simulink model "Yang2011"  (R2019a)
settings: Solver=VariableStepAuto  StartTime=0.0  StopTime=tsim  MaxStep=1e-3  RelTol=1e-12  EnableMultiTasking=on
values from neighbouring files (symbols this model uses):
  A = [a11 a12 0;a21 0 a23;0 a32 0]    [aa_MAGLEV_changeSlope.m]
  Ap = 0.01    [aa_MAGLEV_changeSlope.m]
  B1 = eye(3)    [aa_MAGLEV_changeSlope.m]
  B2 = [b2_11;0;0]    [aa_MAGLEV_changeSlope.m]
  G0 = 0.015    [aa_MAGLEV_changeSlope.m]
  I0 = (1/Kb)*B0*G0    [aa_MAGLEV_changeSlope.m]
  Kb = 0.0015    [aa_MAGLEV_changeSlope.m]
  KdY = -inv([0 0 1]*inv(A+B2*Kx)*B2)*[0 0 1]*inv(A+B2*Kx)*B1    [aa_MAGLEV_changeSlope.m]
  Kf = 9810    [aa_MAGLEV_changeSlope.m]
  KxY = Kx    [aa_MAGLEV_changeSlope.m]
  Lc = 0.1    [aa_MAGLEV_changeSlope.m]
  LY = [40 0 0 ... (first row only)    [aa_MAGLEV_changeSlope.m]
  mc = 1000    [aa_MAGLEV_changeSlope.m]
  Nc = 2000    [aa_MAGLEV_changeSlope.m]
  Rc = 10    [aa_MAGLEV_changeSlope.m]
  V0 = I0*Rc    [aa_MAGLEV_changeSlope.m]
settings Model: Creator=alcasfra  LastModifiedBy=alcas
settings SolverCC: AlgebraicLoopSolver=LineSearch
settings DataIOCC: ReturnWorkspaceOutputs=off
settings OptimizationCC: LifeSpan=inf
settings DebuggingCC: SFUnexpectedBacktrackingDiag=warning  SFNoUnconditionalDefaultTransitionDiag=warning  ArithmeticOperatorsInVariantConditions=warning
settings SFSimCC: SimUseLocalCustomCode=off
settings RTWCC: RTWUseLocalCustomCode=off
settings CodeAppCC: StateflowObjectComments=on
settings GRTTargetCC: TargetLangStandard=C89/C90 (ANSI)  GeneratePreprocessorConditionals=Disable all
settings ConfigComp: CovMetricSettings=dw  CovHtmlReporting=on  CovSaveCumulativeToWorkspaceVar=on  CovSaveSingleToWorkspaceVar=on  CovExternalEMLEnable=off

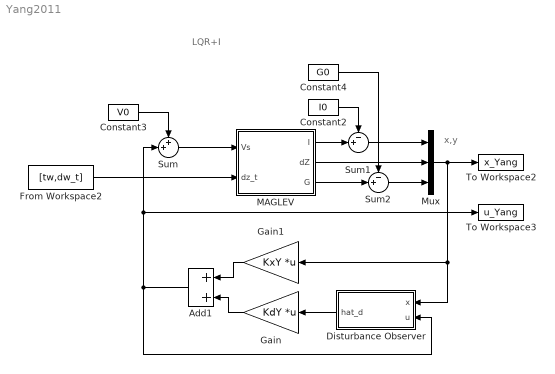
== system Yang2011 ==
  note: x,y
  note: LQR+I
  Add1 : Sum
  Constant2 : Constant  Value=I0
  Constant3 : Constant  Value=V0
  Constant4 : Constant  Value=G0
  Disturbance Observer : Subsystem
  From Workspace2 : FromWorkspace  VariableName=[tw,dw_t]  SampleTime=0
  Gain : Gain  Gain=KdY  Multiplication=Matrix(K*u)
  Gain1 : Gain  Gain=KxY  Multiplication=Matrix(K*u)
  MAGLEV : Subsystem
  Mux : Mux  Inputs=3
  Sum : Sum  Inputs=++|
  Sum1 : Sum  Inputs=-+|
  Sum2 : Sum  Inputs=-+|
  To Workspace2 : ToWorkspace  VariableName=x_Yang  SaveFormat=Structure With Time  SampleTime=-1
  To Workspace3 : ToWorkspace  VariableName=u_Yang  SaveFormat=Structure With Time  SampleTime=-1
  wires:
  Sum/1 -> MAGLEV/1(Vs)
  Constant3/1 -> Sum/1
  MAGLEV/1(I) -> Sum1/2
  Sum1/1 -> Mux/1
  MAGLEV/3(G) -> Sum2/2
  Sum2/1 -> Mux/3
  Constant2/1 -> Sum1/1
  Constant4/1 -> Sum2/1
  MAGLEV/2(dZ) -> Mux/2
  Mux/1 -> To Workspace2/1, Gain1/1, Disturbance Observer/1(x)
  Disturbance Observer/1(hat_d) -> Gain/1
  Gain1/1 -> Add1/1
  Gain/1 -> Add1/2
  Add1/1 -> Disturbance Observer/2(u), To Workspace3/1, Sum/2
  From Workspace2/1 -> MAGLEV/2(dz_t)

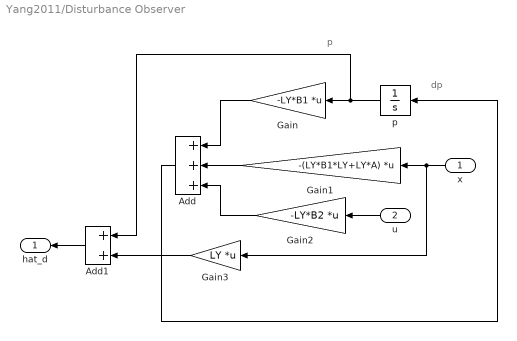
== system Yang2011/Disturbance Observer ==
  note: p
  note: dp
  x : Inport
  u : Inport  Port=2
  Add : Sum  Inputs=+++
  Add1 : Sum
  Gain : Gain  Gain=-LY*B1  Multiplication=Matrix(K*u)
  Gain1 : Gain  Gain=-(LY*B1*LY+LY*A)  Multiplication=Matrix(K*u)
  Gain2 : Gain  Gain=-LY*B2  Multiplication=Matrix(K*u)
  Gain3 : Gain  Gain=LY  Multiplication=Matrix(K*u)
  p : Integrator
  hat_d : Outport
  wires:
  x/1 -> Gain3/1, Gain1/1
  Gain2/1 -> Add/3
  u/1 -> Gain2/1
  Gain3/1 -> Add1/2
  Add1/1 -> hat_d/1
  Add/1 -> p/1
  Gain1/1 -> Add/2
  p/1 -> Add1/1, Gain/1
  Gain/1 -> Add/1

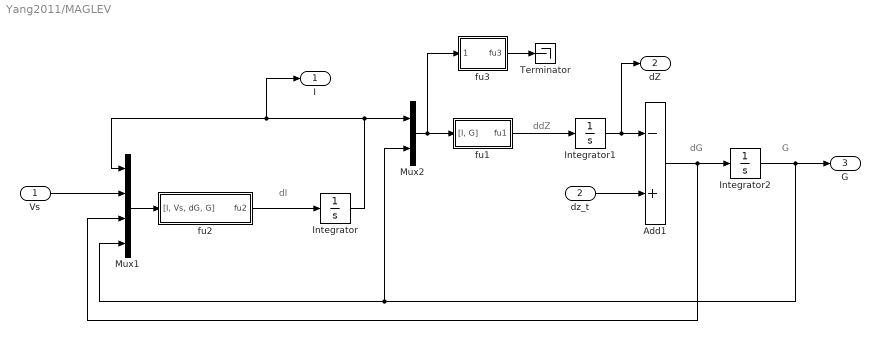
== system Yang2011/MAGLEV ==
  note: G
  note: dG
  note: ddZ
  note: dI
  Vs : Inport
  dz_t : Inport  Port=2
  Add1 : Sum  Inputs=-+
  Integrator : Integrator  InitialCondition=I0
  Integrator1 : Integrator
  Integrator2 : Integrator  InitialCondition=G0
  Mux1 : Mux
  Mux2 : Mux  Inputs=2
  Terminator : Terminator
  fu1 : Subsystem
  fu2 : Subsystem
  fu3 : Subsystem
  I : Outport
  dZ : Outport  Port=2
  G : Outport  Port=3
  wires:
  fu3/1(fu3) -> Terminator/1
  Integrator/1 -> Mux2/1, I/1, Mux1/1
  fu1/1(fu1) -> Integrator1/1
  Integrator2/1 -> Mux2/2, Mux1/4, G/1
  Add1/1 -> Mux1/3, Integrator2/1
  dz_t/1 -> Add1/2
  Integrator1/1 -> dZ/1, Add1/1
  Mux2/1 -> fu3/1("[I, G]"), fu1/1("[I, G]")
  fu2/1(fu2) -> Integrator/1
  Mux1/1 -> fu2/1("[I, Vs, dG, G]")
  Vs/1 -> Mux1/2

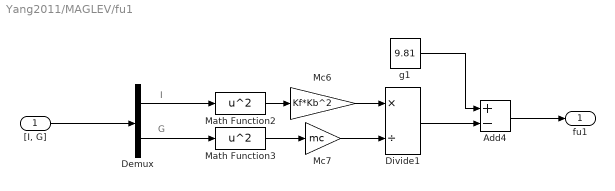
== system Yang2011/MAGLEV/fu1 ==
  note: G
  note: I
  "[I, G]" : Inport
  Add4 : Sum  Inputs=+-
  Demux : Demux  Outputs=2
  Divide1 : Product  Inputs=*/
  Math Function2 : Math  Operator=square  SaturateOnIntegerOverflow=on
  Math Function3 : Math  Operator=square  SaturateOnIntegerOverflow=on
  Mc6 : Gain  Gain=Kf*Kb^2
  Mc7 : Gain  Gain=mc
  g1 : Constant  Value=9.81
  fu1 : Outport
  wires:
  g1/1 -> Add4/1
  Math Function2/1 -> Mc6/1
  Add4/1 -> fu1/1
  Demux/2 -> Math Function3/1
  "[I, G]"/1 -> Demux/1
  Demux/1 -> Math Function2/1
  Divide1/1 -> Add4/2
  Math Function3/1 -> Mc7/1
  Mc7/1 -> Divide1/2
  Mc6/1 -> Divide1/1

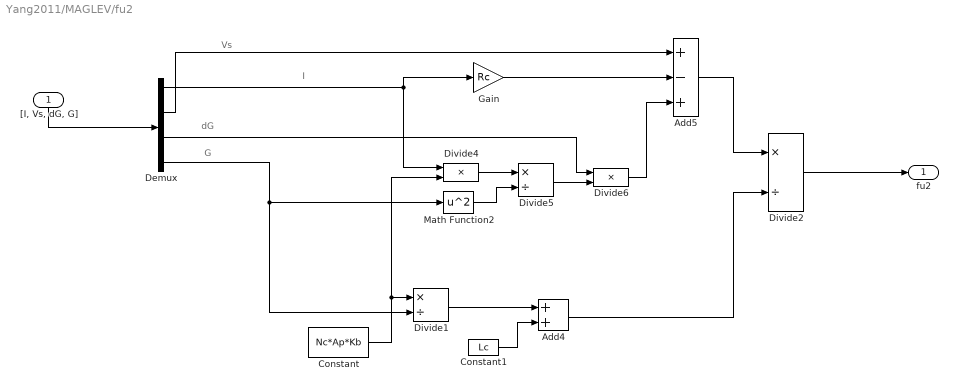
== system Yang2011/MAGLEV/fu2 ==
  note: G
  note: dG
  note: Vs
  note: I
  "[I, Vs, dG, G]" : Inport
  Add4 : Sum
  Add5 : Sum  Inputs=+-+
  Constant : Constant  Value=Nc*Ap*Kb
  Constant1 : Constant  Value=Lc
  Demux : Demux
  Divide1 : Product  Inputs=*/
  Divide2 : Product  Inputs=*/
  Divide4 : Product  Inputs=**
  Divide5 : Product  Inputs=*/
  Divide6 : Product  Inputs=**
  Gain : Gain  Gain=Rc
  Math Function2 : Math  Operator=square  SaturateOnIntegerOverflow=on
  fu2 : Outport
  wires:
  Demux/1 -> Gain/1, Divide4/1
  Constant/1 -> Divide4/2, Divide1/1
  Divide2/1 -> fu2/1
  Constant1/1 -> Add4/2
  Demux/2 -> Add5/1
  Add5/1 -> Divide2/1
  Demux/4 -> Divide1/2, Math Function2/1
  Demux/3 -> Divide6/1
  "[I, Vs, dG, G]"/1 -> Demux/1
  Divide5/1 -> Divide6/2
  Divide1/1 -> Add4/1
  Add4/1 -> Divide2/2
  Math Function2/1 -> Divide5/2
  Divide4/1 -> Divide5/1
  Divide6/1 -> Add5/3
  Gain/1 -> Add5/2

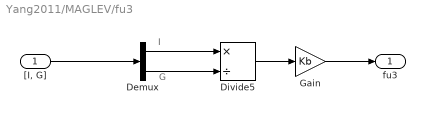
== system Yang2011/MAGLEV/fu3 ==
  note: G
  note: I
  "[I, G]" : Inport
  Demux : Demux  Outputs=2
  Divide5 : Product  Inputs=*/
  Gain : Gain  Gain=Kb
  fu3 : Outport
  wires:
  Demux/2 -> Divide5/2
  Demux/1 -> Divide5/1
  Gain/1 -> fu3/1
  "[I, G]"/1 -> Demux/1
  Divide5/1 -> Gain/1
